simulink model "threephaseinverter_mosfet_model"  (R2026a)
settings: Solver=VariableStepAuto  StopTime=0.3
undefined symbols (not defined in the file): fout, fsw, ModIndex, Rload, Vg
libraries: fl_lib x41, nesl_utility x37, ee_lib x10, simulink x1
(part 1 of 2)
settings Model: Creator=walmy  LastModifiedBy=walmy
settings SimscapeCC: SimscapeNominalValues="[{\"value\":\"1\",\"unit\":\"A\"},{\"value\":\"1\",\"unit\":\"bar\"},{\"value\":\"1\",\"unit\":\"cm^2\"},{\"value\":\"1\",\"unit\":\"cm^3/s\"},{\"value\":\"1\",\"unit\":\"kJ/kg\"},{\"value\":\"1\",\"unit\":\"kW\"},{\"value\":\"1\",\"unit\":\"l\"},{\"value\":\"1\",\"unit\":\"N\"},{\"value\":\"1\",\"unit\":\"N*m\"},{\"value\":\"1\",\"unit\":\"V\"}]"  SimscapeLogType=none  SimscapeLogDataHistory=5000.0

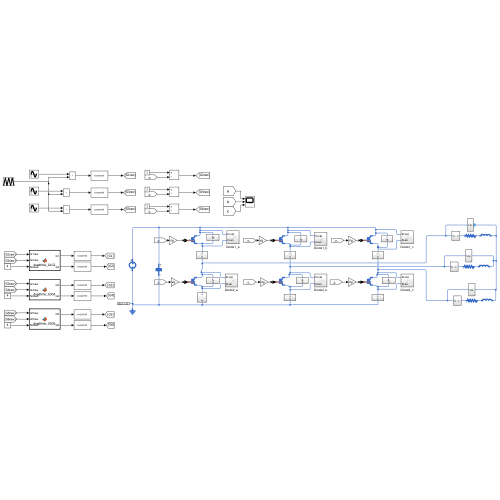
[thumbnail: Simulink's stored preview of the top-level diagram]
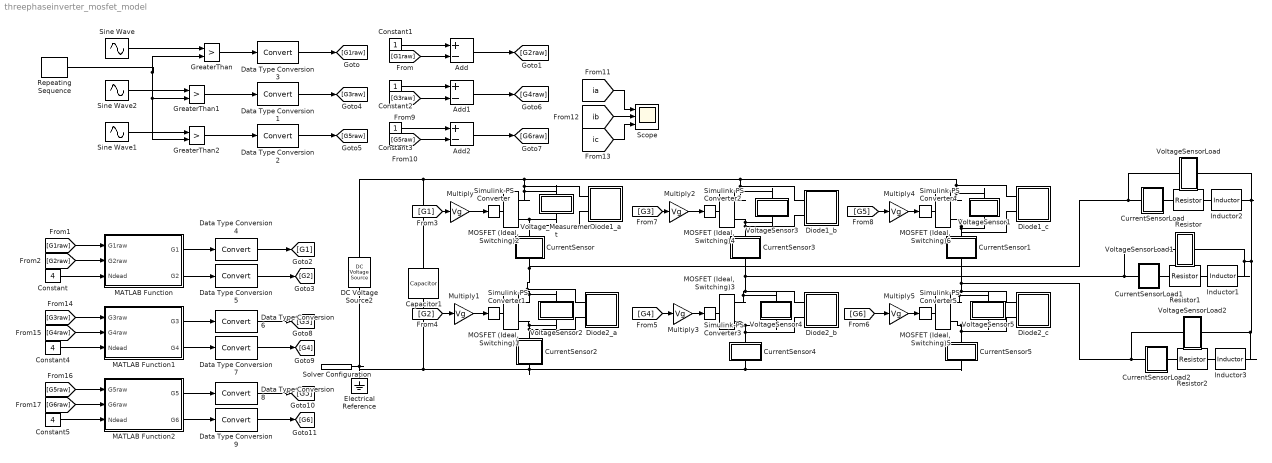
== system threephaseinverter_mosfet_model ==
  Add : Sum  Inputs=+-
  Add1 : Sum  Inputs=+-
  Add2 : Sum  Inputs=+-
  Capacitor1 : fl_lib/Electrical/Electrical Elements/Capacitor  c=Cdc F  r=1e-6 Ohm  g=0 1/Ohm  i_specify=off  i_priority=None  i=0 A  i_nominal_specify=off  i_nominal_value=1  i_nominal_unit=A  v_specify=off  v_priority=None  v=0 V  v_nominal_specify=off  v_nominal_value=1  v_nominal_unit=V  vc_specify=off  vc_priority=High  vc=0 V  vc_nominal_specify=off  vc_nominal_value=1  vc_nominal_unit=V
  Constant : Constant  Value=4
  Constant1 : Constant
  Constant2 : Constant
  Constant3 : Constant
  Constant4 : Constant  Value=4
  Constant5 : Constant  Value=4
  CurrentSensor : Subsystem
  CurrentSensor1 : Subsystem
  CurrentSensor2 : Subsystem
  CurrentSensor3 : Subsystem
  CurrentSensor4 : Subsystem
  CurrentSensor5 : Subsystem
  CurrentSensorLoad : Subsystem
  CurrentSensorLoad1 : Subsystem
  CurrentSensorLoad2 : Subsystem
  DC Voltage Source2 : ee_lib/Additional Components/SPICE Sources/DC Voltage Source  DC=Vdc V
  Data Type Conversion{1..9} (9 alike) : DataTypeConversion  SaturateOnIntegerOverflow=off  RndMeth=Floor
  Diode1_a : Subsystem
  Diode1_b : Subsystem
  Diode1_c : Subsystem
  Diode2_a : Subsystem
  Diode2_b : Subsystem
  Diode2_c : Subsystem
  Electrical Reference : fl_lib/Electrical/Electrical Elements/Electrical Reference
  GreaterThan : RelationalOperator  Operator=>  OutDataTypeStr=boolean  RndMeth=Simplest  InputSameDT=off
  GreaterThan1 : RelationalOperator  Operator=>  OutDataTypeStr=boolean  RndMeth=Simplest  InputSameDT=off
  GreaterThan2 : RelationalOperator  Operator=>  OutDataTypeStr=boolean  RndMeth=Simplest  InputSameDT=off
  Inductor1 : ee_lib/Passive/Inductor  l=Lload H  enable_L_tol=ee.enum.toleranceApplication.none  L_tol=20  tol_distribution=ee.enum.toleranceDistribution.uniform  nSigma=4  r=0 Ohm  g=1e-9 1/Ohm  enable_operating_limits=ee.enum.enable.no  operating_limit_action=ee.enum.passive.reportOpLim.warn  max_working_current=1 A  power_rating=1 W  i_L_specify=off  i_L_priority=High  i_L=0 A  i_L_nominal_specify=off  i_L_nominal_value=1  i_L_nominal_unit=A
  Inductor2 : ee_lib/Passive/Inductor  l=Lload H  enable_L_tol=ee.enum.toleranceApplication.none  L_tol=20  tol_distribution=ee.enum.toleranceDistribution.uniform  nSigma=4  r=0 Ohm  g=1e-9 1/Ohm  enable_operating_limits=ee.enum.enable.no  operating_limit_action=ee.enum.passive.reportOpLim.warn  max_working_current=1 A  power_rating=1 W  i_L_specify=off  i_L_priority=High  i_L=0 A  i_L_nominal_specify=off  i_L_nominal_value=1  i_L_nominal_unit=A
  Inductor3 : ee_lib/Passive/Inductor  l=Lload H  enable_L_tol=ee.enum.toleranceApplication.none  L_tol=20  tol_distribution=ee.enum.toleranceDistribution.uniform  nSigma=4  r=0 Ohm  g=1e-9 1/Ohm  enable_operating_limits=ee.enum.enable.no  operating_limit_action=ee.enum.passive.reportOpLim.warn  max_working_current=1 A  power_rating=1 W  i_L_specify=off  i_L_priority=High  i_L=0 A  i_L_nominal_specify=off  i_L_nominal_value=1  i_L_nominal_unit=A
  MATLAB Function : MATLAB Function  TreatAsAtomicUnit=on
  MATLAB Function1 : MATLAB Function  TreatAsAtomicUnit=on
  MATLAB Function2 : MATLAB Function  TreatAsAtomicUnit=on
  MOSFET (Ideal, Switching){1..6} (6 alike) : ee_lib/Semiconductors & Converters/MOSFET (Ideal, Switching)  port_option=ee.enum.controlport.ps  Rds=RdsOn Ohm  Goff=1e-6 1/Ohm  Vth=2 V  diode_param=ee.enum.semiconductors.protectionDiode.external  diode_Vf=0 V  diode_Ron=0 Ohm  diode_Goff=0 1/Ohm  diode_C=50e-9 F  diode_iRM=-235 A  diode_iF=300 A  diode_idot=-50 A/us  diode_trr_param=ee.enum.converters.diodeReverseParam.trr_factor  diode_trr_factor=3  diode_trr=15 us  diode_Qrr=1500 s*uA  ids_specify=off  ids_priority=None  ids=0 A  ids_nominal_specify=off  ids_nominal_value=1  ids_nominal_unit=A  vds_specify=off  vds_priority=None  vds=0 V  vds_nominal_specify=off  vds_nominal_value=1  vds_nominal_unit=V  vgs_specify=off  vgs_priority=None  vgs=0 V  vgs_nominal_specify=off  vgs_nominal_value=1  vgs_nominal_unit=V  thermal_loss_option=ee.enum.converters.thermalLossOption.constantvalues  Von_data=[0, 1.8, 3.2, 6, 10, 16; 0, 2, 5.5, 9.5, 15, 25] V  Tj=[298.15, 448.15] K  Iout_data=[0, 20, 40, 60, 80, 100] A  tabulateWithVds=false  Eon_data=[0, 55.04, 124.57, 235.53, 362.12; 0, 71.25, 161.25, 304.88, 468.75] * 1e-6 J  Eoff_data=[0, 18, 30, 56.1, 76.5; 0, 22.5, 37.5, 70.13, 95.63] * 1e-6 J  Eon_data_3D=[zeros(2, 5, 3)] J  Eoff_data_3D=[zeros(2, 5, 3)] J  Tj_loss=[298.15, 448.15] K  Iout_data_loss=[0, 10, 20, 30, 40] A  Vds_loss=[0, 150, 300] V  Eon_scalar=22.86e-3 J  Eoff_scalar=17.14e-3 J  Voff=300 V  Iout_scalar=600 A  useCurrentFromPreviousCycle=false  useVoltageFromPreviousCycle=false  diodeModelType=ee.enum.converters.diodeModelType.pwl  diodeTableType=ee.enum.diode.tableType.IfMat  diode_ReverseIVType=ee.enum.diode.diodeReverseIV.constant  diode_IfMat=[.07, .12, .19, 1.75, 4.24, 7.32, 11.2; .16, .3, .72, 2.14, 4.02, 6.35, 9.12] A  diode_VfMat=[.9, 1.15, 1.25, 1.5, 1.75, 2.17, 2.6, 2.85; .58, .68, .75, 1.1, 1.38, 1.77, 2.27, 2.7] V  diode_TjVec=[25, 125] degC  diode_VfVec=[.5, .7, .9, 1.3, 1.7, 2.1, 2.5] V  diode_IfVec=[.1, .2, .5, 1, 2, 4, 7, 10] A  diode_IrMat=[1e-06, 2e-06, 5e-06, 1e-05, 2.5e-05, 5e-05, .0001; 2e-06, 5e-06, 1e-05, 4e-05, 8e-05, .0002, .0005] A  diode_VrMat=[10, 100, 200, 250, 300, 325, 350; 10, 70, 160, 220, 270, 300, 320] V  diode_VrVec=[10, 20, 40, 50, 70, 80, 100] V  diode_IrVec=[1e-06, 2e-06, 5e-06, 1e-05, 2e-05, 5e-05, .0001] A  diode_Vr=-600 V  diode_Ls=150 nH  diode_Erec=0.03 J  diode_rec_loss_model=ee.enum.diode.reverseRecoveryModel.fixed  diode_ErecVal=0 J  diode_scaleWithIandV=true  diode_ErecMat=zeros(2, 3) J  diodeErecMat3D=zeros(2, 3, 2) J  diode_TjrecVec=[298.15, 398.15] K  diode_IfrecVec=[.1, 1, 10] A  diodeVrecVec=[0, 100] V  diode_IrecVal=10 A  diode_VrecVal=10 V  diode_tFilter=1 / 1000 / 100 s  separateThermalPortForDiode=false  thermal_network_parameterization=ee.enum.thermalNetworkTopology.external  Rth=[.03, .2] K/W  Rth_Cauer=[.03, .1, .2] K/W  Rth_Foster=[.08, .14, .22, .16] K/W  thermal_mass_parameterization=ee.enum.thermalNetwork.timeconstant  thermal_mass=[3, 25] J/K  thermal_mass_Cauer=[3, 10, 25] J/K  thermal_mass_Foster=[.001, .005, .05, .5] J/K  thermal_time_constant=[.1, 5] s  thermal_time_constant_Cauer=[.1, 1, 5] s  thermal_time_constant_Foster=[7e-05, .0007, .01, .08] s  thermal_mass_initial_temperatures=[25, 25] degC  thermal_mass_initial_temperatures_Cauer=[25, 25, 25] degC  junction_thermal_mass=0.1 J/K  Tvec_initial_Foster=[25, 25, 25, 25] degC  RthDiode=[.03, .2] K/W  RthCauerDiode=[.03, .1, .2] K/W  RthFosterDiode=[.03, .2] K/W  thermalMassDiode=[3, 25] J/K  thermalMassCauerDiode=[3, 10, 25] J/K  thermalMassFosterDiode=[33, 50] J/K  thermalTauDiode=[.1, 5] s  thermalTauCauerDiode=[.1, 1, 5] s  thermalTauFosterDiode=[1, 10] s  thermalMassInitTempDiode=[25, 25] degC  thermalMassInitTempCauerDiode=[25, 25, 25] degC  junctionthermalMassDiode=0.1 J/K  TVecInitialFosterDiode=[25, 25, 25, 25] degC  no_thermal_network=0  mosfet_junction_temperature_specify=off  mosfet_junction_temperature_priority=None  mosfet_junction_temperature=25 degC  mosfet_junction_temperature_nominal_specify=off  mosfet_junction_temperature_nominal_value=1  mosfet_junction_temperature_nominal_unit=degC  diode_junction_temperature_specify=off  diode_junction_temperature_priority=None  diode_junction_temperature=25 degC  diode_junction_temperature_nominal_specify=off  diode_junction_temperature_nominal_value=1  diode_junction_temperature_nominal_unit=degC  Qj_specify=off  Qj_priority=None  Qj=0 W  Qj_nominal_specify=off  Qj_nominal_value=1  Qj_nominal_unit=W  accumulatedSwitchingLosses_specify=off  accumulatedSwitchingLosses_priority=None  accumulatedSwitchingLosses=0 J
  Multiply{,1..5} (6 alike) : Gain  Gain=Vg
  Repeating Sequence : simulink/Sources/Repeating Sequence  rep_seq_t=[0 1/(2*fsw) 1/fsw]  rep_seq_y=[-1 1 -1]
  Resistor : fl_lib/Electrical/Electrical Elements/Resistor  R=Rload Ohm  i_specify=off  i_priority=None  i=0 A  i_nominal_specify=off  i_nominal_value=1  i_nominal_unit=A  v_specify=off  v_priority=None  v=0 V  v_nominal_specify=off  v_nominal_value=1  v_nominal_unit=V
  Resistor1 : fl_lib/Electrical/Electrical Elements/Resistor  R=Rload Ohm  i_specify=off  i_priority=None  i=0 A  i_nominal_specify=off  i_nominal_value=1  i_nominal_unit=A  v_specify=off  v_priority=None  v=0 V  v_nominal_specify=off  v_nominal_value=1  v_nominal_unit=V
  Resistor2 : fl_lib/Electrical/Electrical Elements/Resistor  R=Rload Ohm  i_specify=off  i_priority=None  i=0 A  i_nominal_specify=off  i_nominal_value=1  i_nominal_unit=A  v_specify=off  v_priority=None  v=0 V  v_nominal_specify=off  v_nominal_value=1  v_nominal_unit=V
  Scope : Scope  NumInputPorts=3
      settings: ActiveDisplayYMinimum=-13.763418111566516  ActiveDisplayYMaximum=13.269695362503114  DataLoggingVariableName=ScopeData2
  Simulink-PS Converter{,1..5} (6 alike) : nesl_utility/Simulink-PS Converter  PhysicalDomain=network_engine_domain  SubClassName=ps_input  LeftPortType=input  RightPortType=output  PseudoPeriodic=off  Frequencies=[]  NoiseDistribution=none  NoiseParameters=[]  Unit=1  AffineConversion=off  FilteringAndDerivatives=provide  SimscapeFilterOrder=1  InputFilterTimeConstant=0.001  UdotUserProvided=0
  Sine Wave : Sin  Amplitude=ModIndex  Frequency=2*pi*fout  SampleTime=0
  Sine Wave1 : Sin  Amplitude=ModIndex  Frequency=2*pi*fout  Phase=2*pi/3  SampleTime=0
  Sine Wave2 : Sin  Amplitude=ModIndex  Frequency=2*pi*fout  Phase=-2*pi/3  SampleTime=0
  Solver Configuration : nesl_utility/Solver Configuration  PhysicalDomain=network_engine_domain  SubClassName=solver  LeftPortType=input  RightPortType=generic  Tones=[]  Harmonics=[]  SimulateNoise=off  Profile=off  UseLocalSampling=off  EnableSwitchedLinearOptims=on  FrequencyDomain=off  UseCCode=off  RelTol=0.001  AbsTol=0.001  MinStep=1e-09  ToWorkspace=off  RevertToSquareIcSolve=off  NumHomotopyIterations=100  PhasorMode=off  PhasorModeNumHarmonics=1  ConsistencySolver=NEWTON_XTOL_AFTER_FTOL  CanonicalOrdering=UNORDERED  OptimizeIntermediates=UNOPTIMIZED  IndexReductionMethod=DerivativeReplacement  DoDC=off  ResidualTolerance=1e-09  ConsistencyTolSource=GLOBAL  ConsistencyAbsTol=0.001  ConsistencyRelTol=0.001  ConsistencyTolFactor=0.001  UseLocalSolver=on  LocalSolverChoice=NE_BACKWARD_EULER_ADVANCER  ResolveIndetEquations=on  FunctionEvalNumThread=1  LocalSolverSampleTime=1e-6  DoFixedCost=off  MaxNonlinIter=3  MaxModeIter=2  ComputeImpulses=off  ImpulseIterations=2  LinearAlgebra=auto  LinearAlgebraNumThread=0  EquationFormulation=NE_TIME_EF  DelaysMemoryBudget=1024  AutomaticFiltering=on  FilteringTimeConstant=0.001  PartitionStorageMethod=AS_NEEDED  PartitionMemoryBudget=1024  PartitionMethod=ROBUST  MultibodyUseLocalSolver=off  MultibodyLocalSolverChoice=ODE1  MultibodyLocalSolverSampleTime=0.001
  VoltageSensor1 : Subsystem
  VoltageSensor2 : Subsystem
  VoltageSensor3 : Subsystem
  VoltageSensor4 : Subsystem
  VoltageSensor5 : Subsystem
  VoltageSensorLoad : Subsystem
  VoltageSensorLoad1 : Subsystem
  VoltageSensorLoad2 : Subsystem
  Voltage_Measurement : Subsystem
  wires:
  [G1raw] -> MATLAB Function/1(G1raw)
  [G2raw] -> MATLAB Function/2(G2raw)
  Constant/1 -> MATLAB Function/3(Ndead)
  MATLAB Function/1(G1) -> Data Type Conversion4/1
  MATLAB Function/2(G2) -> Data Type Conversion5/1
  [G1] -> Multiply/1
  Multiply3/1 -> Simulink-PS Converter3/1
  Multiply2/1 -> Simulink-PS Converter2/1
  [G1raw] -> Add/2
  Add/1 -> [G2raw]
  Data Type Conversion3/1 -> [G1raw]
  Sine Wave/1 -> GreaterThan/1
  Constant1/1 -> Add/1
  Repeating Sequence/1 -> GreaterThan2/2, GreaterThan1/2, GreaterThan/2
  GreaterThan/1 -> Data Type Conversion3/1
  Multiply/1 -> Simulink-PS Converter/1
  Multiply1/1 -> Simulink-PS Converter1/1
  [G2] -> Multiply1/1
  [G3] -> Multiply2/1
  [G4] -> Multiply3/1
  [G6] -> Multiply5/1
  [G5] -> Multiply4/1
  Multiply4/1 -> Simulink-PS Converter4/1
  Multiply5/1 -> Simulink-PS Converter5/1
  Sine Wave2/1 -> GreaterThan1/1
  Sine Wave1/1 -> GreaterThan2/1
  GreaterThan1/1 -> Data Type Conversion1/1
  GreaterThan2/1 -> Data Type Conversion2/1
  Data Type Conversion1/1 -> [G3raw]
  Data Type Conversion2/1 -> [G5raw]
  Constant2/1 -> Add1/1
  Add1/1 -> [G4raw]
  [G3raw] -> Add1/2
  [G5raw] -> Add2/2
  Add2/1 -> [G6raw]
  Constant3/1 -> Add2/1
  [ia] -> Scope/1
  [ib] -> Scope/2
  [ic] -> Scope/3
  MATLAB Function1/2(G4) -> Data Type Conversion7/1
  MATLAB Function1/1(G3) -> Data Type Conversion6/1
  Constant4/1 -> MATLAB Function1/3(Ndead)
  [G4raw] -> MATLAB Function1/2(G4raw)
  [G3raw] -> MATLAB Function1/1(G3raw)
  [G5raw] -> MATLAB Function2/1(G5raw)
  [G6raw] -> MATLAB Function2/2(G6raw)
  Constant5/1 -> MATLAB Function2/3(Ndead)
  MATLAB Function2/1(G5) -> Data Type Conversion8/1
  MATLAB Function2/2(G6) -> Data Type Conversion9/1
  Data Type Conversion4/1 -> [G1]
  Data Type Conversion5/1 -> [G2]
  Data Type Conversion6/1 -> [G3]
  Data Type Conversion7/1 -> [G4]
  Data Type Conversion8/1 -> [G5]
  Data Type Conversion9/1 -> [G6]
  connections:
  "MOSFET (Ideal, Switching)2"/RConn2 -- Diode1_a/LConn2 -- CurrentSensor/RConn1 -- Voltage_Measurement/RConn1
  Simulink-PS Converter/RConn1 -- "MOSFET (Ideal, Switching)2"/LConn1
  Simulink-PS Converter1/RConn1 -- "MOSFET (Ideal, Switching)1"/LConn1
  "MOSFET (Ideal, Switching)4"/RConn2 -- Diode1_b/LConn2 -- CurrentSensor3/RConn1 -- VoltageSensor3/RConn1
  VoltageSensor4/RConn1 -- Diode2_b/LConn2 -- CurrentSensor4/RConn1 -- "MOSFET (Ideal, Switching)3"/RConn2
  Simulink-PS Converter2/RConn1 -- "MOSFET (Ideal, Switching)4"/LConn1
  Simulink-PS Converter3/RConn1 -- "MOSFET (Ideal, Switching)3"/LConn1
  Solver Configuration/RConn1 -- CurrentSensor5/LConn1 -- CurrentSensor4/LConn1 -- CurrentSensor2/LConn1 -- Capacitor1/RConn1 -- Electrical Reference/LConn1 -- DC Voltage Source2/RConn1
  "MOSFET (Ideal, Switching)1"/RConn2 -- Diode2_a/LConn2 -- CurrentSensor2/RConn1 -- VoltageSensor2/RConn1
  Diode1_c/LConn1 -- "MOSFET (Ideal, Switching)6"/RConn1 -- VoltageSensor1/LConn1 -- Diode1_b/LConn1 -- "MOSFET (Ideal, Switching)4"/RConn1 -- VoltageSensor3/LConn1 -- Diode1_a/LConn1 -- "MOSFET (Ideal, Switching)2"/RConn1 -- Voltage_Measurement/LConn1 -- DC Voltage Source2/LConn1 -- Capacitor1/LConn1
  CurrentSensor/LConn1 -- VoltageSensorLoad/LConn1 -- CurrentSensorLoad/LConn1 -- Diode2_a/LConn1 -- "MOSFET (Ideal, Switching)1"/RConn1 -- VoltageSensor2/LConn1
  Resistor/LConn1 -- Inductor2/LConn1
  CurrentSensorLoad/RConn1 -- Resistor/RConn1
  VoltageSensor1/RConn1 -- "MOSFET (Ideal, Switching)6"/RConn2 -- CurrentSensor1/RConn1 -- Diode1_c/LConn2
  Diode2_c/LConn2 -- CurrentSensor5/RConn1 -- "MOSFET (Ideal, Switching)5"/RConn2 -- VoltageSensor5/RConn1
  Simulink-PS Converter5/RConn1 -- "MOSFET (Ideal, Switching)5"/LConn1
  Simulink-PS Converter4/RConn1 -- "MOSFET (Ideal, Switching)6"/LConn1
  CurrentSensorLoad1/RConn1 -- Resistor1/RConn1
  Resistor1/LConn1 -- Inductor1/LConn1
  Diode2_b/LConn1 -- CurrentSensor3/LConn1 -- CurrentSensorLoad1/LConn1 -- VoltageSensorLoad1/LConn1 -- VoltageSensor4/LConn1 -- "MOSFET (Ideal, Switching)3"/RConn1
  Inductor1/RConn1 -- VoltageSensorLoad/RConn1 -- Inductor2/RConn1 -- Inductor3/RConn1 -- VoltageSensorLoad2/RConn1 -- VoltageSensorLoad1/RConn1
  CurrentSensor1/LConn1 -- Diode2_c/LConn1 -- "MOSFET (Ideal, Switching)5"/RConn1 -- VoltageSensor5/LConn1 -- VoltageSensorLoad2/LConn1 -- CurrentSensorLoad2/LConn1
  Resistor2/LConn1 -- Inductor3/LConn1
  CurrentSensorLoad2/RConn1 -- Resistor2/RConn1

== system threephaseinverter_mosfet_model/CurrentSensor ==
  Current Sensor4 : fl_lib/Electrical/Electrical Sensors/Current Sensor
  PS-Simulink Converter2 : nesl_utility/PS-Simulink Converter  PhysicalDomain=network_engine_domain  SubClassName=ps_output  LeftPortType=input  RightPortType=output  PseudoPeriodic=off  Frequencies=[]  VectorFormat=inherit  Unit=inherit  AffineConversion=off
  To Workspace4 : ToWorkspace  VariableName=Isw1_sim  SaveFormat=Timeseries  SampleTime=-1
  i- : PMIOPort  Side=Right
  i+ : PMIOPort  Port=2  Side=Left
  wires:
  PS-Simulink Converter2/1 -> To Workspace4/1
  connections:
  Current Sensor4/LConn1 -- i+/RConn1
  PS-Simulink Converter2/LConn1 -- Current Sensor4/RConn1
  i-/RConn1 -- Current Sensor4/RConn2

== system threephaseinverter_mosfet_model/CurrentSensor1 ==
  Current Sensor2 : fl_lib/Electrical/Electrical Sensors/Current Sensor
  PS-Simulink Converter2 : nesl_utility/PS-Simulink Converter  PhysicalDomain=network_engine_domain  SubClassName=ps_output  LeftPortType=input  RightPortType=output  PseudoPeriodic=off  Frequencies=[]  VectorFormat=inherit  Unit=inherit  AffineConversion=off
  To Workspace4 : ToWorkspace  VariableName=Isw5_sim  SaveFormat=Timeseries  SampleTime=-1
  i- : PMIOPort  Side=Right
  i+ : PMIOPort  Port=2  Side=Left
  wires:
  PS-Simulink Converter2/1 -> To Workspace4/1
  connections:
  Current Sensor2/LConn1 -- i+/RConn1
  i-/RConn1 -- Current Sensor2/RConn2
  PS-Simulink Converter2/LConn1 -- Current Sensor2/RConn1

== system threephaseinverter_mosfet_model/CurrentSensor2 ==
  Current Sensor5 : fl_lib/Electrical/Electrical Sensors/Current Sensor
  PS-Simulink Converter2 : nesl_utility/PS-Simulink Converter  PhysicalDomain=network_engine_domain  SubClassName=ps_output  LeftPortType=input  RightPortType=output  PseudoPeriodic=off  Frequencies=[]  VectorFormat=inherit  Unit=inherit  AffineConversion=off
  To Workspace4 : ToWorkspace  VariableName=Isw2_sim  SaveFormat=Timeseries  SampleTime=-1
  i- : PMIOPort  Side=Right
  i+ : PMIOPort  Port=2  Side=Left
  wires:
  PS-Simulink Converter2/1 -> To Workspace4/1
  connections:
  PS-Simulink Converter2/LConn1 -- Current Sensor5/RConn1
  Current Sensor5/LConn1 -- i+/RConn1
  Current Sensor5/RConn2 -- i-/RConn1

== system threephaseinverter_mosfet_model/CurrentSensor3 ==
  Current Sensor2 : fl_lib/Electrical/Electrical Sensors/Current Sensor
  PS-Simulink Converter2 : nesl_utility/PS-Simulink Converter  PhysicalDomain=network_engine_domain  SubClassName=ps_output  LeftPortType=input  RightPortType=output  PseudoPeriodic=off  Frequencies=[]  VectorFormat=inherit  Unit=inherit  AffineConversion=off
  To Workspace4 : ToWorkspace  VariableName=Isw3_sim  SaveFormat=Timeseries  SampleTime=-1
  i- : PMIOPort  Side=Right
  i+ : PMIOPort  Port=2  Side=Left
  wires:
  PS-Simulink Converter2/1 -> To Workspace4/1
  connections:
  PS-Simulink Converter2/LConn1 -- Current Sensor2/RConn1
  i-/RConn1 -- Current Sensor2/RConn2
  Current Sensor2/LConn1 -- i+/RConn1

== system threephaseinverter_mosfet_model/CurrentSensor4 ==
  Current Sensor3 : fl_lib/Electrical/Electrical Sensors/Current Sensor
  PS-Simulink Converter2 : nesl_utility/PS-Simulink Converter  PhysicalDomain=network_engine_domain  SubClassName=ps_output  LeftPortType=input  RightPortType=output  PseudoPeriodic=off  Frequencies=[]  VectorFormat=inherit  Unit=inherit  AffineConversion=off
  To Workspace4 : ToWorkspace  VariableName=Isw4_sim  SaveFormat=Timeseries  SampleTime=-1
  i- : PMIOPort  Side=Right
  i+ : PMIOPort  Port=2  Side=Left
  wires:
  PS-Simulink Converter2/1 -> To Workspace4/1
  connections:
  PS-Simulink Converter2/LConn1 -- Current Sensor3/RConn1
  Current Sensor3/LConn1 -- i+/RConn1
  Current Sensor3/RConn2 -- i-/RConn1

== system threephaseinverter_mosfet_model/CurrentSensor5 ==
  Current Sensor3 : fl_lib/Electrical/Electrical Sensors/Current Sensor
  PS-Simulink Converter2 : nesl_utility/PS-Simulink Converter  PhysicalDomain=network_engine_domain  SubClassName=ps_output  LeftPortType=input  RightPortType=output  PseudoPeriodic=off  Frequencies=[]  VectorFormat=inherit  Unit=inherit  AffineConversion=off
  To Workspace4 : ToWorkspace  VariableName=Isw6_sim  SaveFormat=Timeseries  SampleTime=-1
  i- : PMIOPort  Side=Right
  i+ : PMIOPort  Port=2  Side=Left
  wires:
  PS-Simulink Converter2/1 -> To Workspace4/1
  connections:
  Current Sensor3/RConn2 -- i-/RConn1
  Current Sensor3/LConn1 -- i+/RConn1
  PS-Simulink Converter2/LConn1 -- Current Sensor3/RConn1

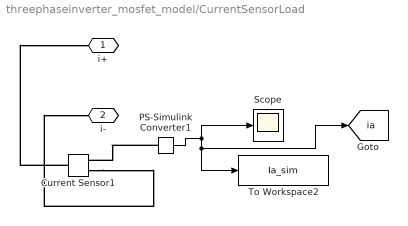
== system threephaseinverter_mosfet_model/CurrentSensorLoad ==
  Current Sensor1 : fl_lib/Electrical/Electrical Sensors/Current Sensor
  PS-Simulink Converter1 : nesl_utility/PS-Simulink Converter  PhysicalDomain=network_engine_domain  SubClassName=ps_output  LeftPortType=input  RightPortType=output  PseudoPeriodic=off  Frequencies=[]  VectorFormat=inherit  Unit=inherit  AffineConversion=off
  Scope : Scope
      settings: ActiveDisplayYMinimum=-38.557663897821215  ActiveDisplayYMaximum=36.363133455666528
  To Workspace2 : ToWorkspace  VariableName=Ia_sim  SaveFormat=Timeseries  SampleTime=-1
  i+ : PMIOPort  Side=Left
  i- : PMIOPort  Port=2  Side=Right
  tag scope: ia=global
  wires:
  PS-Simulink Converter1/1 -> Scope/1, To Workspace2/1, [ia]
  connections:
  PS-Simulink Converter1/LConn1 -- Current Sensor1/RConn1
  Current Sensor1/LConn1 -- i+/RConn1
  Current Sensor1/RConn2 -- i-/RConn1

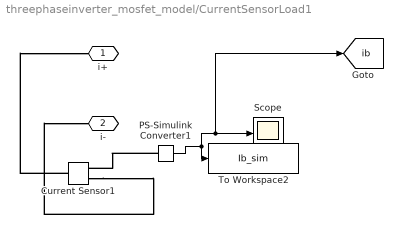
== system threephaseinverter_mosfet_model/CurrentSensorLoad1 ==
  Current Sensor1 : fl_lib/Electrical/Electrical Sensors/Current Sensor
  PS-Simulink Converter1 : nesl_utility/PS-Simulink Converter  PhysicalDomain=network_engine_domain  SubClassName=ps_output  LeftPortType=input  RightPortType=output  PseudoPeriodic=off  Frequencies=[]  VectorFormat=inherit  Unit=inherit  AffineConversion=off
  Scope : Scope
      settings: ActiveDisplayYMinimum=-38.557663897821215  ActiveDisplayYMaximum=36.363133455666528
  To Workspace2 : ToWorkspace  VariableName=Ib_sim  SaveFormat=Timeseries  SampleTime=-1
  i+ : PMIOPort  Side=Left
  i- : PMIOPort  Port=2  Side=Right
  tag scope: ib=global
  wires:
  PS-Simulink Converter1/1 -> [ib], Scope/1, To Workspace2/1
  connections:
  Current Sensor1/RConn2 -- i-/RConn1
  Current Sensor1/LConn1 -- i+/RConn1
  PS-Simulink Converter1/LConn1 -- Current Sensor1/RConn1

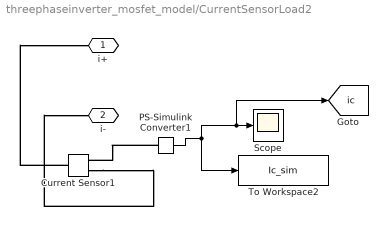
== system threephaseinverter_mosfet_model/CurrentSensorLoad2 ==
  Current Sensor1 : fl_lib/Electrical/Electrical Sensors/Current Sensor
  PS-Simulink Converter1 : nesl_utility/PS-Simulink Converter  PhysicalDomain=network_engine_domain  SubClassName=ps_output  LeftPortType=input  RightPortType=output  PseudoPeriodic=off  Frequencies=[]  VectorFormat=inherit  Unit=inherit  AffineConversion=off
  Scope : Scope
      settings: ActiveDisplayYMinimum=-38.557663897821215  ActiveDisplayYMaximum=36.363133455666528
  To Workspace2 : ToWorkspace  VariableName=Ic_sim  SaveFormat=Timeseries  SampleTime=-1
  i+ : PMIOPort  Side=Left
  i- : PMIOPort  Port=2  Side=Right
  tag scope: ic=global
  wires:
  PS-Simulink Converter1/1 -> [ic], Scope/1, To Workspace2/1
  connections:
  PS-Simulink Converter1/LConn1 -- Current Sensor1/RConn1
  Current Sensor1/LConn1 -- i+/RConn1
  Current Sensor1/RConn2 -- i-/RConn1

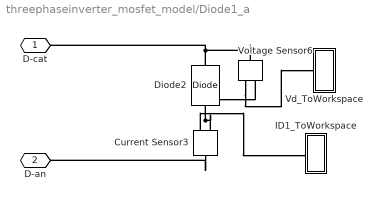
== system threephaseinverter_mosfet_model/Diode1_a ==
  Current Sensor3 : fl_lib/Electrical/Electrical Sensors/Current Sensor
  Diode2 : fl_lib/Electrical/Electrical Elements/Diode  Vf=Vf V  Ron=RonD Ohm  Goff=1e-8 1/Ohm  i_specify=off  i_priority=None  i=0 A  i_nominal_specify=off  i_nominal_value=1  i_nominal_unit=A  v_specify=off  v_priority=None  v=0 V  v_nominal_specify=off  v_nominal_value=1  v_nominal_unit=V
  ID1_ToWorkspace : Subsystem
      settings: PortSchema="{\"entries\":[{\"content\":{\"sides\":[{\"content\":{},\"type\":\"ConnectorPlacement.EquallySpacedRectSide\",\"uuid\":\"27aaa4b5-bd60-4d70-86e5-bc47b9bf8e53\"},{\"content\":{\"side\":\"RIGHT\"},\"type\":\"ConnectorPlacement.EquallySpacedRectSide\",\"uuid\":\"05934d8e-d6a5-4e4d-8439-d59dc6cd6ba8\"},{\"content\":{\"side\":\"TOP\"},\"type\":\"ConnectorPlacement.EquallySpacedRectSide\",\"uuid\":\"aced43fe-b59e-458d-8f58-35c4c9cdeb93\"},{\"content\":{\"connectorIds\":[\"RConn1\"],\"side\":\"BOTTOM\"},\"type\":\"ConnectorPlacement.EquallySpacedRectSide\",\"uuid\":\"aab3351d-4a00-4793-a207-44be8bae81b0\"}]},\"type\":\"ConnectorPlacement.EquallySpacedConnector\",\"uuid\":\"dcaf3857-8a00-4c3d-a0e7-096efad9ae0c\"}],\"packageUris\":[\"http://schema.mathworks.com/mf0/Connector/R2020b\"],\"version\":\"1.0\"}"
  Vd_ToWorkspace : Subsystem
      settings: PortSchema="{\"entries\":[{\"content\":{\"sides\":[{\"content\":{},\"type\":\"ConnectorPlacement.EquallySpacedRectSide\",\"uuid\":\"43f18de1-9718-4cbd-927a-ce7ec8f86ca1\"},{\"content\":{\"side\":\"RIGHT\"},\"type\":\"ConnectorPlacement.EquallySpacedRectSide\",\"uuid\":\"f671083a-78f6-4bee-900b-3feb52f79cdd\"},{\"content\":{\"side\":\"TOP\"},\"type\":\"ConnectorPlacement.EquallySpacedRectSide\",\"uuid\":\"024a9ce1-31bc-419f-b1bc-225b332881fb\"},{\"content\":{\"connectorIds\":[\"RConn1\"],\"side\":\"BOTTOM\"},\"type\":\"ConnectorPlacement.EquallySpacedRectSide\",\"uuid\":\"061c0d43-51f1-4fe9-9216-5b022de32a74\"}]},\"type\":\"ConnectorPlacement.EquallySpacedConnector\",\"uuid\":\"db5cc1c5-1d7d-4018-9977-3b4cf7cfcf03\"}],\"packageUris\":[\"http://schema.mathworks.com/mf0/Connector/R2020b\"],\"version\":\"1.0\"}"
  Voltage Sensor6 : fl_lib/Electrical/Electrical Sensors/Voltage Sensor
  D-cat : PMIOPort  Side=Left
  D-an : PMIOPort  Port=2  Side=Left
  connections:
  Current Sensor3/RConn2 -- Voltage Sensor6/RConn2 -- Diode2/LConn1
  Current Sensor3/RConn1 -- ID1_ToWorkspace/RConn1
  Diode2/RConn1 -- D-cat/RConn1 -- Voltage Sensor6/LConn1
  Voltage Sensor6/RConn1 -- Vd_ToWorkspace/RConn1
  Current Sensor3/LConn1 -- D-an/RConn1

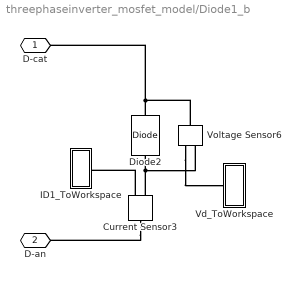
== system threephaseinverter_mosfet_model/Diode1_b ==
  Current Sensor3 : fl_lib/Electrical/Electrical Sensors/Current Sensor
  Diode2 : fl_lib/Electrical/Electrical Elements/Diode  Vf=Vf V  Ron=RonD Ohm  Goff=1e-8 1/Ohm  i_specify=off  i_priority=None  i=0 A  i_nominal_specify=off  i_nominal_value=1  i_nominal_unit=A  v_specify=off  v_priority=None  v=0 V  v_nominal_specify=off  v_nominal_value=1  v_nominal_unit=V
  ID1_ToWorkspace : Subsystem
      settings: PortSchema="{\"entries\":[{\"content\":{\"sides\":[{\"content\":{},\"type\":\"ConnectorPlacement.EquallySpacedRectSide\",\"uuid\":\"27aaa4b5-bd60-4d70-86e5-bc47b9bf8e53\"},{\"content\":{\"side\":\"RIGHT\"},\"type\":\"ConnectorPlacement.EquallySpacedRectSide\",\"uuid\":\"05934d8e-d6a5-4e4d-8439-d59dc6cd6ba8\"},{\"content\":{\"side\":\"TOP\"},\"type\":\"ConnectorPlacement.EquallySpacedRectSide\",\"uuid\":\"aced43fe-b59e-458d-8f58-35c4c9cdeb93\"},{\"content\":{\"connectorIds\":[\"RConn1\"],\"side\":\"BOTTOM\"},\"type\":\"ConnectorPlacement.EquallySpacedRectSide\",\"uuid\":\"aab3351d-4a00-4793-a207-44be8bae81b0\"}]},\"type\":\"ConnectorPlacement.EquallySpacedConnector\",\"uuid\":\"dcaf3857-8a00-4c3d-a0e7-096efad9ae0c\"}],\"packageUris\":[\"http://schema.mathworks.com/mf0/Connector/R2020b\"],\"version\":\"1.0\"}"
  Vd_ToWorkspace : Subsystem
      settings: PortSchema="{\"entries\":[{\"content\":{\"sides\":[{\"content\":{},\"type\":\"ConnectorPlacement.EquallySpacedRectSide\",\"uuid\":\"43f18de1-9718-4cbd-927a-ce7ec8f86ca1\"},{\"content\":{\"side\":\"RIGHT\"},\"type\":\"ConnectorPlacement.EquallySpacedRectSide\",\"uuid\":\"f671083a-78f6-4bee-900b-3feb52f79cdd\"},{\"content\":{\"side\":\"TOP\"},\"type\":\"ConnectorPlacement.EquallySpacedRectSide\",\"uuid\":\"024a9ce1-31bc-419f-b1bc-225b332881fb\"},{\"content\":{\"connectorIds\":[\"RConn1\"],\"side\":\"BOTTOM\"},\"type\":\"ConnectorPlacement.EquallySpacedRectSide\",\"uuid\":\"061c0d43-51f1-4fe9-9216-5b022de32a74\"}]},\"type\":\"ConnectorPlacement.EquallySpacedConnector\",\"uuid\":\"db5cc1c5-1d7d-4018-9977-3b4cf7cfcf03\"}],\"packageUris\":[\"http://schema.mathworks.com/mf0/Connector/R2020b\"],\"version\":\"1.0\"}"
  Voltage Sensor6 : fl_lib/Electrical/Electrical Sensors/Voltage Sensor
  D-cat : PMIOPort  Side=Left
  D-an : PMIOPort  Port=2  Side=Left
  connections:
  Current Sensor3/RConn2 -- Voltage Sensor6/RConn2 -- Diode2/LConn1
  Current Sensor3/RConn1 -- ID1_ToWorkspace/RConn1
  Voltage Sensor6/LConn1 -- D-cat/RConn1 -- Diode2/RConn1
  Voltage Sensor6/RConn1 -- Vd_ToWorkspace/RConn1
  Current Sensor3/LConn1 -- D-an/RConn1

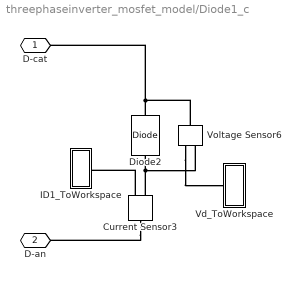
== system threephaseinverter_mosfet_model/Diode1_c ==
  Current Sensor3 : fl_lib/Electrical/Electrical Sensors/Current Sensor
  Diode2 : fl_lib/Electrical/Electrical Elements/Diode  Vf=Vf V  Ron=RonD Ohm  Goff=1e-8 1/Ohm  i_specify=off  i_priority=None  i=0 A  i_nominal_specify=off  i_nominal_value=1  i_nominal_unit=A  v_specify=off  v_priority=None  v=0 V  v_nominal_specify=off  v_nominal_value=1  v_nominal_unit=V
  ID1_ToWorkspace : Subsystem
      settings: PortSchema="{\"entries\":[{\"content\":{\"sides\":[{\"content\":{},\"type\":\"ConnectorPlacement.EquallySpacedRectSide\",\"uuid\":\"27aaa4b5-bd60-4d70-86e5-bc47b9bf8e53\"},{\"content\":{\"side\":\"RIGHT\"},\"type\":\"ConnectorPlacement.EquallySpacedRectSide\",\"uuid\":\"05934d8e-d6a5-4e4d-8439-d59dc6cd6ba8\"},{\"content\":{\"side\":\"TOP\"},\"type\":\"ConnectorPlacement.EquallySpacedRectSide\",\"uuid\":\"aced43fe-b59e-458d-8f58-35c4c9cdeb93\"},{\"content\":{\"connectorIds\":[\"RConn1\"],\"side\":\"BOTTOM\"},\"type\":\"ConnectorPlacement.EquallySpacedRectSide\",\"uuid\":\"aab3351d-4a00-4793-a207-44be8bae81b0\"}]},\"type\":\"ConnectorPlacement.EquallySpacedConnector\",\"uuid\":\"dcaf3857-8a00-4c3d-a0e7-096efad9ae0c\"}],\"packageUris\":[\"http://schema.mathworks.com/mf0/Connector/R2020b\"],\"version\":\"1.0\"}"
  Vd_ToWorkspace : Subsystem
      settings: PortSchema="{\"entries\":[{\"content\":{\"sides\":[{\"content\":{},\"type\":\"ConnectorPlacement.EquallySpacedRectSide\",\"uuid\":\"43f18de1-9718-4cbd-927a-ce7ec8f86ca1\"},{\"content\":{\"side\":\"RIGHT\"},\"type\":\"ConnectorPlacement.EquallySpacedRectSide\",\"uuid\":\"f671083a-78f6-4bee-900b-3feb52f79cdd\"},{\"content\":{\"side\":\"TOP\"},\"type\":\"ConnectorPlacement.EquallySpacedRectSide\",\"uuid\":\"024a9ce1-31bc-419f-b1bc-225b332881fb\"},{\"content\":{\"connectorIds\":[\"RConn1\"],\"side\":\"BOTTOM\"},\"type\":\"ConnectorPlacement.EquallySpacedRectSide\",\"uuid\":\"061c0d43-51f1-4fe9-9216-5b022de32a74\"}]},\"type\":\"ConnectorPlacement.EquallySpacedConnector\",\"uuid\":\"db5cc1c5-1d7d-4018-9977-3b4cf7cfcf03\"}],\"packageUris\":[\"http://schema.mathworks.com/mf0/Connector/R2020b\"],\"version\":\"1.0\"}"
  Voltage Sensor6 : fl_lib/Electrical/Electrical Sensors/Voltage Sensor
  D-cat : PMIOPort  Side=Left
  D-an : PMIOPort  Port=2  Side=Left
  connections:
  Current Sensor3/LConn1 -- D-an/RConn1
  Voltage Sensor6/RConn1 -- Vd_ToWorkspace/RConn1
  Diode2/RConn1 -- D-cat/RConn1 -- Voltage Sensor6/LConn1
  Current Sensor3/RConn1 -- ID1_ToWorkspace/RConn1
  Diode2/LConn1 -- Voltage Sensor6/RConn2 -- Current Sensor3/RConn2

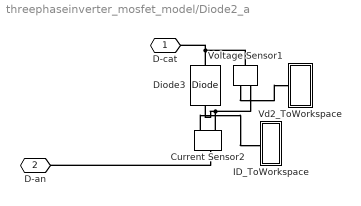
== system threephaseinverter_mosfet_model/Diode2_a ==
  Current Sensor2 : fl_lib/Electrical/Electrical Sensors/Current Sensor
  Diode3 : fl_lib/Electrical/Electrical Elements/Diode  Vf=Vf V  Ron=RonD Ohm  Goff=1e-8 1/Ohm  i_specify=off  i_priority=None  i=0 A  i_nominal_specify=off  i_nominal_value=1  i_nominal_unit=A  v_specify=off  v_priority=None  v=0 V  v_nominal_specify=off  v_nominal_value=1  v_nominal_unit=V
  ID_ToWorkspace : Subsystem
      settings: PortSchema="{\"entries\":[{\"content\":{\"sides\":[{\"content\":{},\"type\":\"ConnectorPlacement.EquallySpacedRectSide\",\"uuid\":\"5b175078-bf36-45f4-9d6d-54820150d16a\"},{\"content\":{\"side\":\"RIGHT\"},\"type\":\"ConnectorPlacement.EquallySpacedRectSide\",\"uuid\":\"3e3920a0-040e-4405-9234-56971fc67e62\"},{\"content\":{\"connectorIds\":[\"LConn1\"],\"side\":\"TOP\"},\"type\":\"ConnectorPlacement.EquallySpacedRectSide\",\"uuid\":\"d1eeb1f1-e8ae-4d22-bde1-4e1f65563d0c\"}]},\"type\":\"ConnectorPlacement.EquallySpacedConnector\",\"uuid\":\"fd63cd4a-cbe3-4add-a632-837285ffcc78\"}],\"packageUris\":[\"http://schema.mathworks.com/mf0/Connector/R2020b\"],\"version\":\"1.0\"}"
  Vd2_ToWorkspace : Subsystem
  Voltage Sensor1 : fl_lib/Electrical/Electrical Sensors/Voltage Sensor
  D-cat : PMIOPort  Side=Left
  D-an : PMIOPort  Port=2  Side=Left
  connections:
  Diode3/RConn1 -- D-cat/RConn1 -- Voltage Sensor1/LConn1
  Voltage Sensor1/RConn1 -- Vd2_ToWorkspace/LConn1
  Current Sensor2/RConn2 -- Voltage Sensor1/RConn2 -- Diode3/LConn1
  Current Sensor2/LConn1 -- D-an/RConn1
  Current Sensor2/RConn1 -- ID_ToWorkspace/LConn1

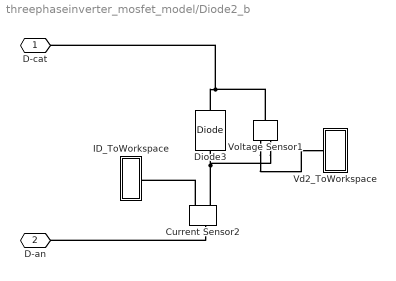
== system threephaseinverter_mosfet_model/Diode2_b ==
  Current Sensor2 : fl_lib/Electrical/Electrical Sensors/Current Sensor
  Diode3 : fl_lib/Electrical/Electrical Elements/Diode  Vf=Vf V  Ron=RonD Ohm  Goff=1e-8 1/Ohm  i_specify=off  i_priority=None  i=0 A  i_nominal_specify=off  i_nominal_value=1  i_nominal_unit=A  v_specify=off  v_priority=None  v=0 V  v_nominal_specify=off  v_nominal_value=1  v_nominal_unit=V
  ID_ToWorkspace : Subsystem
      settings: PortSchema="{\"entries\":[{\"content\":{\"sides\":[{\"content\":{},\"type\":\"ConnectorPlacement.EquallySpacedRectSide\",\"uuid\":\"5b175078-bf36-45f4-9d6d-54820150d16a\"},{\"content\":{\"side\":\"RIGHT\"},\"type\":\"ConnectorPlacement.EquallySpacedRectSide\",\"uuid\":\"3e3920a0-040e-4405-9234-56971fc67e62\"},{\"content\":{\"connectorIds\":[\"LConn1\"],\"side\":\"TOP\"},\"type\":\"ConnectorPlacement.EquallySpacedRectSide\",\"uuid\":\"d1eeb1f1-e8ae-4d22-bde1-4e1f65563d0c\"}]},\"type\":\"ConnectorPlacement.EquallySpacedConnector\",\"uuid\":\"fd63cd4a-cbe3-4add-a632-837285ffcc78\"}],\"packageUris\":[\"http://schema.mathworks.com/mf0/Connector/R2020b\"],\"version\":\"1.0\"}"
  Vd2_ToWorkspace : Subsystem
  Voltage Sensor1 : fl_lib/Electrical/Electrical Sensors/Voltage Sensor
  D-cat : PMIOPort  Side=Left
  D-an : PMIOPort  Port=2  Side=Left
  connections:
  Voltage Sensor1/LConn1 -- Diode3/RConn1 -- D-cat/RConn1
  Voltage Sensor1/RConn1 -- Vd2_ToWorkspace/LConn1
  Voltage Sensor1/RConn2 -- Current Sensor2/RConn2 -- Diode3/LConn1
  Current Sensor2/LConn1 -- D-an/RConn1
  Current Sensor2/RConn1 -- ID_ToWorkspace/LConn1

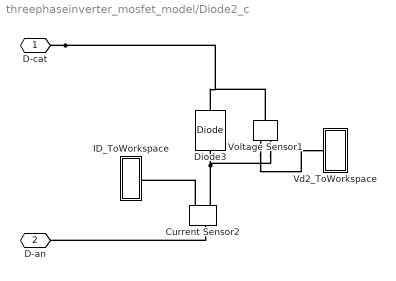
== system threephaseinverter_mosfet_model/Diode2_c ==
  Current Sensor2 : fl_lib/Electrical/Electrical Sensors/Current Sensor
  Diode3 : fl_lib/Electrical/Electrical Elements/Diode  Vf=Vf V  Ron=RonD Ohm  Goff=1e-8 1/Ohm  i_specify=off  i_priority=None  i=0 A  i_nominal_specify=off  i_nominal_value=1  i_nominal_unit=A  v_specify=off  v_priority=None  v=0 V  v_nominal_specify=off  v_nominal_value=1  v_nominal_unit=V
  ID_ToWorkspace : Subsystem
      settings: PortSchema="{\"entries\":[{\"content\":{\"sides\":[{\"content\":{},\"type\":\"ConnectorPlacement.EquallySpacedRectSide\",\"uuid\":\"5b175078-bf36-45f4-9d6d-54820150d16a\"},{\"content\":{\"side\":\"RIGHT\"},\"type\":\"ConnectorPlacement.EquallySpacedRectSide\",\"uuid\":\"3e3920a0-040e-4405-9234-56971fc67e62\"},{\"content\":{\"connectorIds\":[\"LConn1\"],\"side\":\"TOP\"},\"type\":\"ConnectorPlacement.EquallySpacedRectSide\",\"uuid\":\"d1eeb1f1-e8ae-4d22-bde1-4e1f65563d0c\"}]},\"type\":\"ConnectorPlacement.EquallySpacedConnector\",\"uuid\":\"fd63cd4a-cbe3-4add-a632-837285ffcc78\"}],\"packageUris\":[\"http://schema.mathworks.com/mf0/Connector/R2020b\"],\"version\":\"1.0\"}"
  Vd2_ToWorkspace : Subsystem
  Voltage Sensor1 : fl_lib/Electrical/Electrical Sensors/Voltage Sensor
  D-cat : PMIOPort  Side=Left
  D-an : PMIOPort  Port=2  Side=Left
  connections:
  Current Sensor2/RConn1 -- ID_ToWorkspace/LConn1
  Current Sensor2/LConn1 -- D-an/RConn1
  Diode3/LConn1 -- Current Sensor2/RConn2 -- Voltage Sensor1/RConn2
  Voltage Sensor1/RConn1 -- Vd2_ToWorkspace/LConn1
  D-cat/RConn1 -- Diode3/RConn1 -- Voltage Sensor1/LConn1

== system threephaseinverter_mosfet_model/VoltageSensor1 ==
  PS-Simulink Converter1 : nesl_utility/PS-Simulink Converter  PhysicalDomain=network_engine_domain  SubClassName=ps_output  LeftPortType=input  RightPortType=output  PseudoPeriodic=off  Frequencies=[]  VectorFormat=inherit  Unit=inherit  AffineConversion=off
  To Workspace12 : ToWorkspace  VariableName=VDS5_sim  SaveFormat=Timeseries  SampleTime=-1
  Voltage Sensor1 : fl_lib/Electrical/Electrical Sensors/Voltage Sensor
  v+ : PMIOPort  Side=Left
  v- : PMIOPort  Port=2  Side=Right
  wires:
  PS-Simulink Converter1/1 -> To Workspace12/1
  connections:
  Voltage Sensor1/RConn2 -- v-/RConn1
  PS-Simulink Converter1/LConn1 -- Voltage Sensor1/RConn1
  Voltage Sensor1/LConn1 -- v+/RConn1

== system threephaseinverter_mosfet_model/VoltageSensor2 ==
  PS-Simulink Converter2 : nesl_utility/PS-Simulink Converter  PhysicalDomain=network_engine_domain  SubClassName=ps_output  LeftPortType=input  RightPortType=output  PseudoPeriodic=off  Frequencies=[]  VectorFormat=inherit  Unit=inherit  AffineConversion=off
  To Workspace12 : ToWorkspace  VariableName=VDS2_sim  SaveFormat=Timeseries  SampleTime=-1
  Voltage Sensor4 : fl_lib/Electrical/Electrical Sensors/Voltage Sensor
  v+ : PMIOPort  Side=Left
  v- : PMIOPort  Port=2  Side=Right
  wires:
  PS-Simulink Converter2/1 -> To Workspace12/1
  connections:
  PS-Simulink Converter2/LConn1 -- Voltage Sensor4/RConn1
  Voltage Sensor4/LConn1 -- v+/RConn1
  Voltage Sensor4/RConn2 -- v-/RConn1

== system threephaseinverter_mosfet_model/VoltageSensor3 ==
  PS-Simulink Converter1 : nesl_utility/PS-Simulink Converter  PhysicalDomain=network_engine_domain  SubClassName=ps_output  LeftPortType=input  RightPortType=output  PseudoPeriodic=off  Frequencies=[]  VectorFormat=inherit  Unit=inherit  AffineConversion=off
  To Workspace12 : ToWorkspace  VariableName=VDS3_sim  SaveFormat=Timeseries  SampleTime=-1
  Voltage Sensor1 : fl_lib/Electrical/Electrical Sensors/Voltage Sensor
  v+ : PMIOPort  Side=Left
  v- : PMIOPort  Port=2  Side=Right
  wires:
  PS-Simulink Converter1/1 -> To Workspace12/1
  connections:
  Voltage Sensor1/LConn1 -- v+/RConn1
  PS-Simulink Converter1/LConn1 -- Voltage Sensor1/RConn1
  Voltage Sensor1/RConn2 -- v-/RConn1

== system threephaseinverter_mosfet_model/VoltageSensor4 ==
  PS-Simulink Converter2 : nesl_utility/PS-Simulink Converter  PhysicalDomain=network_engine_domain  SubClassName=ps_output  LeftPortType=input  RightPortType=output  PseudoPeriodic=off  Frequencies=[]  VectorFormat=inherit  Unit=inherit  AffineConversion=off
  To Workspace12 : ToWorkspace  VariableName=VDS4_sim  SaveFormat=Timeseries  SampleTime=-1
  Voltage Sensor5 : fl_lib/Electrical/Electrical Sensors/Voltage Sensor
  v+ : PMIOPort  Side=Left
  v- : PMIOPort  Port=2  Side=Right
  wires:
  PS-Simulink Converter2/1 -> To Workspace12/1
  connections:
  PS-Simulink Converter2/LConn1 -- Voltage Sensor5/RConn1
  Voltage Sensor5/LConn1 -- v+/RConn1
  Voltage Sensor5/RConn2 -- v-/RConn1

== system threephaseinverter_mosfet_model/VoltageSensor5 ==
  PS-Simulink Converter2 : nesl_utility/PS-Simulink Converter  PhysicalDomain=network_engine_domain  SubClassName=ps_output  LeftPortType=input  RightPortType=output  PseudoPeriodic=off  Frequencies=[]  VectorFormat=inherit  Unit=inherit  AffineConversion=off
  To Workspace12 : ToWorkspace  VariableName=VDS6_sim  SaveFormat=Timeseries  SampleTime=-1
  Voltage Sensor5 : fl_lib/Electrical/Electrical Sensors/Voltage Sensor
  v+ : PMIOPort  Side=Left
  v- : PMIOPort  Port=2  Side=Right
  wires:
  PS-Simulink Converter2/1 -> To Workspace12/1
  connections:
  Voltage Sensor5/RConn2 -- v-/RConn1
  Voltage Sensor5/LConn1 -- v+/RConn1
  PS-Simulink Converter2/LConn1 -- Voltage Sensor5/RConn1

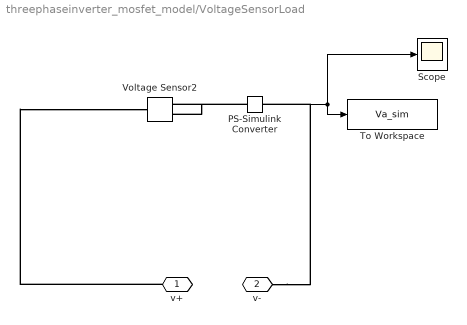
== system threephaseinverter_mosfet_model/VoltageSensorLoad ==
  PS-Simulink Converter : nesl_utility/PS-Simulink Converter  PhysicalDomain=network_engine_domain  SubClassName=ps_output  LeftPortType=input  RightPortType=output  PseudoPeriodic=off  Frequencies=[]  VectorFormat=inherit  Unit=inherit  AffineConversion=off
  Scope : Scope
      settings: ActiveDisplayYMinimum=-583.52571959853981  ActiveDisplayYMaximum=583.27289957288258
  To Workspace : ToWorkspace  VariableName=Va_sim  SaveFormat=Timeseries  SampleTime=-1
  Voltage Sensor2 : fl_lib/Electrical/Electrical Sensors/Voltage Sensor
  v+ : PMIOPort  Side=Left
  v- : PMIOPort  Port=2  Side=Right
  wires:
  PS-Simulink Converter/1 -> Scope/1, To Workspace/1
  connections:
  PS-Simulink Converter/LConn1 -- Voltage Sensor2/RConn1
  v+/RConn1 -- Voltage Sensor2/LConn1
  v-/RConn1 -- Voltage Sensor2/RConn2

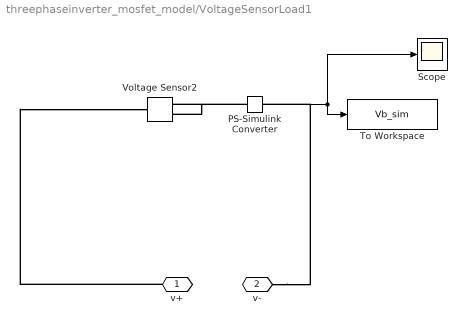
== system threephaseinverter_mosfet_model/VoltageSensorLoad1 ==
  PS-Simulink Converter : nesl_utility/PS-Simulink Converter  PhysicalDomain=network_engine_domain  SubClassName=ps_output  LeftPortType=input  RightPortType=output  PseudoPeriodic=off  Frequencies=[]  VectorFormat=inherit  Unit=inherit  AffineConversion=off
  Scope : Scope
      settings: ActiveDisplayYMinimum=-450.16194300627961  ActiveDisplayYMaximum=51.486652355456883
  To Workspace : ToWorkspace  VariableName=Vb_sim  SaveFormat=Timeseries  SampleTime=-1
  Voltage Sensor2 : fl_lib/Electrical/Electrical Sensors/Voltage Sensor
  v+ : PMIOPort  Side=Left
  v- : PMIOPort  Port=2  Side=Right
  wires:
  PS-Simulink Converter/1 -> To Workspace/1, Scope/1
  connections:
  v-/RConn1 -- Voltage Sensor2/RConn2
  v+/RConn1 -- Voltage Sensor2/LConn1
  PS-Simulink Converter/LConn1 -- Voltage Sensor2/RConn1

== system threephaseinverter_mosfet_model/VoltageSensorLoad2 ==
  PS-Simulink Converter : nesl_utility/PS-Simulink Converter  PhysicalDomain=network_engine_domain  SubClassName=ps_output  LeftPortType=input  RightPortType=output  PseudoPeriodic=off  Frequencies=[]  VectorFormat=inherit  Unit=inherit  AffineConversion=off
  Scope : Scope
      settings: ActiveDisplayYMinimum=-450.16194300627961  ActiveDisplayYMaximum=51.486652355456883
  To Workspace : ToWorkspace  VariableName=Vc_sim  SaveFormat=Timeseries  SampleTime=-1
  Voltage Sensor2 : fl_lib/Electrical/Electrical Sensors/Voltage Sensor
  v+ : PMIOPort  Side=Left
  v- : PMIOPort  Port=2  Side=Right
  wires:
  PS-Simulink Converter/1 -> Scope/1, To Workspace/1
  connections:
  PS-Simulink Converter/LConn1 -- Voltage Sensor2/RConn1
  v+/RConn1 -- Voltage Sensor2/LConn1
  v-/RConn1 -- Voltage Sensor2/RConn2

== system threephaseinverter_mosfet_model/Voltage_Measurement ==
  PS-Simulink Converter1 : nesl_utility/PS-Simulink Converter  PhysicalDomain=network_engine_domain  SubClassName=ps_output  LeftPortType=input  RightPortType=output  PseudoPeriodic=off  Frequencies=[]  VectorFormat=inherit  Unit=inherit  AffineConversion=off
  To Workspace12 : ToWorkspace  VariableName=VDS1_sim  SaveFormat=Timeseries  SampleTime=-1
  Voltage Sensor3 : fl_lib/Electrical/Electrical Sensors/Voltage Sensor
  v+ : PMIOPort  Side=Left
  v- : PMIOPort  Port=2  Side=Right
  wires:
  PS-Simulink Converter1/1 -> To Workspace12/1
  connections:
  Voltage Sensor3/LConn1 -- v+/RConn1
  PS-Simulink Converter1/LConn1 -- Voltage Sensor3/RConn1
  Voltage Sensor3/RConn2 -- v-/RConn1

== system threephaseinverter_mosfet_model/Diode1_a/ID1_ToWorkspace ==
  PS-Simulink Converter1 : nesl_utility/PS-Simulink Converter  PhysicalDomain=network_engine_domain  SubClassName=ps_output  LeftPortType=input  RightPortType=output  PseudoPeriodic=off  Frequencies=[]  VectorFormat=inherit  Unit=inherit  AffineConversion=off
  To Workspace6 : ToWorkspace  VariableName=ID1_sim  SaveFormat=Timeseries  SampleTime=-1
  Conn1 : PMIOPort  Side=Right
  wires:
  PS-Simulink Converter1/1 -> To Workspace6/1
  connections:
  PS-Simulink Converter1/LConn1 -- Conn1/RConn1

== system threephaseinverter_mosfet_model/Diode1_a/Vd_ToWorkspace ==
  PS-Simulink Converter5 : nesl_utility/PS-Simulink Converter  PhysicalDomain=network_engine_domain  SubClassName=ps_output  LeftPortType=input  RightPortType=output  PseudoPeriodic=off  Frequencies=[]  VectorFormat=inherit  Unit=inherit  AffineConversion=off
  To Workspace12 : ToWorkspace  VariableName=VD1_sim  SaveFormat=Timeseries  SampleTime=-1
  y : PMIOPort  Side=Right
  wires:
  PS-Simulink Converter5/1 -> To Workspace12/1
  connections:
  y/RConn1 -- PS-Simulink Converter5/LConn1

== system threephaseinverter_mosfet_model/Diode1_b/ID1_ToWorkspace ==
  PS-Simulink Converter1 : nesl_utility/PS-Simulink Converter  PhysicalDomain=network_engine_domain  SubClassName=ps_output  LeftPortType=input  RightPortType=output  PseudoPeriodic=off  Frequencies=[]  VectorFormat=inherit  Unit=inherit  AffineConversion=off
  To Workspace6 : ToWorkspace  VariableName=ID3_sim  SaveFormat=Timeseries  SampleTime=-1
  Conn1 : PMIOPort  Side=Right
  wires:
  PS-Simulink Converter1/1 -> To Workspace6/1
  connections:
  PS-Simulink Converter1/LConn1 -- Conn1/RConn1

== system threephaseinverter_mosfet_model/Diode1_b/Vd_ToWorkspace ==
  PS-Simulink Converter5 : nesl_utility/PS-Simulink Converter  PhysicalDomain=network_engine_domain  SubClassName=ps_output  LeftPortType=input  RightPortType=output  PseudoPeriodic=off  Frequencies=[]  VectorFormat=inherit  Unit=inherit  AffineConversion=off
  To Workspace12 : ToWorkspace  VariableName=VD3_sim  SaveFormat=Timeseries  SampleTime=-1
  y : PMIOPort  Side=Right
  wires:
  PS-Simulink Converter5/1 -> To Workspace12/1
  connections:
  y/RConn1 -- PS-Simulink Converter5/LConn1

== system threephaseinverter_mosfet_model/Diode1_c/ID1_ToWorkspace ==
  PS-Simulink Converter1 : nesl_utility/PS-Simulink Converter  PhysicalDomain=network_engine_domain  SubClassName=ps_output  LeftPortType=input  RightPortType=output  PseudoPeriodic=off  Frequencies=[]  VectorFormat=inherit  Unit=inherit  AffineConversion=off
  To Workspace6 : ToWorkspace  VariableName=ID5_sim  SaveFormat=Timeseries  SampleTime=-1
  Conn1 : PMIOPort  Side=Right
  wires:
  PS-Simulink Converter1/1 -> To Workspace6/1
  connections:
  PS-Simulink Converter1/LConn1 -- Conn1/RConn1

== system threephaseinverter_mosfet_model/Diode1_c/Vd_ToWorkspace ==
  PS-Simulink Converter5 : nesl_utility/PS-Simulink Converter  PhysicalDomain=network_engine_domain  SubClassName=ps_output  LeftPortType=input  RightPortType=output  PseudoPeriodic=off  Frequencies=[]  VectorFormat=inherit  Unit=inherit  AffineConversion=off
  To Workspace12 : ToWorkspace  VariableName=VD5_sim  SaveFormat=Timeseries  SampleTime=-1
  y : PMIOPort  Side=Right
  wires:
  PS-Simulink Converter5/1 -> To Workspace12/1
  connections:
  y/RConn1 -- PS-Simulink Converter5/LConn1

== system threephaseinverter_mosfet_model/Diode2_a/ID_ToWorkspace ==
  PS-Simulink Converter8 : nesl_utility/PS-Simulink Converter  PhysicalDomain=network_engine_domain  SubClassName=ps_output  LeftPortType=input  RightPortType=output  PseudoPeriodic=off  Frequencies=[]  VectorFormat=inherit  Unit=inherit  AffineConversion=off
  To Workspace6 : ToWorkspace  VariableName=ID2_sim  SaveFormat=Timeseries  SampleTime=-1
  y : PMIOPort  Side=Left
  wires:
  PS-Simulink Converter8/1 -> To Workspace6/1
  connections:
  y/RConn1 -- PS-Simulink Converter8/LConn1

== system threephaseinverter_mosfet_model/Diode2_a/Vd2_ToWorkspace ==
  PS-Simulink Converter7 : nesl_utility/PS-Simulink Converter  PhysicalDomain=network_engine_domain  SubClassName=ps_output  LeftPortType=input  RightPortType=output  PseudoPeriodic=off  Frequencies=[]  VectorFormat=inherit  Unit=inherit  AffineConversion=off
  To Workspace12 : ToWorkspace  VariableName=VD2_sim  SaveFormat=Timeseries  SampleTime=-1
  u : PMIOPort  Side=Left
  wires:
  PS-Simulink Converter7/1 -> To Workspace12/1

== system threephaseinverter_mosfet_model/Diode2_b/ID_ToWorkspace ==
  PS-Simulink Converter8 : nesl_utility/PS-Simulink Converter  PhysicalDomain=network_engine_domain  SubClassName=ps_output  LeftPortType=input  RightPortType=output  PseudoPeriodic=off  Frequencies=[]  VectorFormat=inherit  Unit=inherit  AffineConversion=off
  To Workspace6 : ToWorkspace  VariableName=ID4_sim  SaveFormat=Timeseries  SampleTime=-1
  y : PMIOPort  Side=Left
  wires:
  PS-Simulink Converter8/1 -> To Workspace6/1
  connections:
  y/RConn1 -- PS-Simulink Converter8/LConn1

== system threephaseinverter_mosfet_model/Diode2_b/Vd2_ToWorkspace ==
  PS-Simulink Converter7 : nesl_utility/PS-Simulink Converter  PhysicalDomain=network_engine_domain  SubClassName=ps_output  LeftPortType=input  RightPortType=output  PseudoPeriodic=off  Frequencies=[]  VectorFormat=inherit  Unit=inherit  AffineConversion=off
  To Workspace12 : ToWorkspace  VariableName=VD4_sim  SaveFormat=Timeseries  SampleTime=-1
  u : PMIOPort  Side=Left
  wires:
  PS-Simulink Converter7/1 -> To Workspace12/1
  connections:
  PS-Simulink Converter7/LConn1 -- u/RConn1

== system threephaseinverter_mosfet_model/Diode2_c/ID_ToWorkspace ==
  PS-Simulink Converter8 : nesl_utility/PS-Simulink Converter  PhysicalDomain=network_engine_domain  SubClassName=ps_output  LeftPortType=input  RightPortType=output  PseudoPeriodic=off  Frequencies=[]  VectorFormat=inherit  Unit=inherit  AffineConversion=off
  To Workspace6 : ToWorkspace  VariableName=ID6_sim  SaveFormat=Timeseries  SampleTime=-1
  y : PMIOPort  Side=Left
  wires:
  PS-Simulink Converter8/1 -> To Workspace6/1
  connections:
  y/RConn1 -- PS-Simulink Converter8/LConn1

== system threephaseinverter_mosfet_model/Diode2_c/Vd2_ToWorkspace ==
  PS-Simulink Converter7 : nesl_utility/PS-Simulink Converter  PhysicalDomain=network_engine_domain  SubClassName=ps_output  LeftPortType=input  RightPortType=output  PseudoPeriodic=off  Frequencies=[]  VectorFormat=inherit  Unit=inherit  AffineConversion=off
  To Workspace12 : ToWorkspace  VariableName=VD6_sim  SaveFormat=Timeseries  SampleTime=-1
  u : PMIOPort  Side=Left
  wires:
  PS-Simulink Converter7/1 -> To Workspace12/1
  connections:
  PS-Simulink Converter7/LConn1 -- u/RConn1
